simulink model "ssc_car_fuel_cell_1motor"  (R2026a)
settings: Solver=daessc  StopTime=195  FixedStep=1e-3  AbsTol=1e-3
InitFcn:
  | %Vehicle = sm_car_vehcfg_checkConfig(Vehicle);
undefined symbols (not defined in the file): Control, Driver, Init, Maneuver1, Vehicle
libraries: fl_lib x93, nesl_utility x38, GasN_lib x21, sdl_lib x10, simulink_extras x6, SimscapeFluids_lib x6, simulink x5, customMath_lib x5, slpidlib x4, ee_lib x3, autolibshared x2, sl_discontinuities x2
(part 4 of 4)

== system ssc_car_fuel_cell_1motor/Vehicle/Powertrain/FuelCell1Motor/Fuel Cell/Fuel Cell/Oxygen Source/Humidifier ==
  Desired RH : Inport
  Constant : Constant  Value=FuelCell.Humidifier.Tin.Value
  Filter : Subsystem  mask(First-order lag supporting vector signals){b=[1 1 1 1]*0.01, x_initial=[0 0 0 0]}
      mask prompts: b "Filter time constant"; x_initial "Initial output"
      mask help: Models a lag of the form 1/(b*s+1) where s is the Laplace operator.
  Gain : Gain  Gain=[0;0;0;1]
  PS-Simulink Converter : nesl_utility/PS-Simulink Converter  PhysicalDomain=network_engine_domain  SubClassName=ps_output  LeftPortType=input  RightPortType=output  PseudoPeriodic=off  Frequencies=[]  VectorFormat=1-D array  Unit=1  AffineConversion=off
  Perfect Insulator : fl_lib/Thermal/Thermal Elements/Perfect Insulator  T_specify=off  T_priority=None  T=0 K  T_nominal_specify=off  T_nominal_value=1  T_nominal_unit=K
  Pipe : GasN_lib/Pipe (N Gas)  length=FuelCell.Humidifier.xPipe.Value m  area=FuelCell.Humidifier.areaPipe.Value cm^2  Dh=FuelCell.Humidifier.dHydraulic.Value cm  extra_length=FuelCell.Humidifier.xFriction.Value m  roughness=FuelCell.Humidifier.roughness.Value m  Re_lam=FuelCell.Humidifier.laminarReynoldsMax.Value  Re_tur=FuelCell.Humidifier.turbulentReynoldsMin.Value  shape_factor=FuelCell.Humidifier.frictionDarcy.Value  Nu_lam=FuelCell.Humidifier.laminarNusselt.Value  p0=FuelCell.Humidifier.p.Value MPa  T0=FuelCell.Humidifier.T.Value degC  comp=GasN.composition_enum.mole  y0=FuelCell.Humidifier.rMoleFractions.Value'  x0=[1; 0; 0; 0]  tau_c=FuelCell.Humidifier.timeCondensation.Value s  isCond=FuelCell.Humidifier.speciesCondensed.Value'
  Simulink-PS Converter : nesl_utility/Simulink-PS Converter  PhysicalDomain=network_engine_domain  SubClassName=ps_input  LeftPortType=input  RightPortType=output  PseudoPeriodic=off  Frequencies=[]  NoiseDistribution=none  NoiseParameters=[]  Unit=1  AffineConversion=off  FilteringAndDerivatives=provide  SimscapeFilterOrder=1  InputFilterTimeConstant=0.001  UdotUserProvided=0
  Simulink-PS Converter1 : nesl_utility/Simulink-PS Converter  PhysicalDomain=network_engine_domain  SubClassName=ps_input  LeftPortType=input  RightPortType=output  PseudoPeriodic=off  Frequencies=[]  NoiseDistribution=none  NoiseParameters=[]  Unit=1  AffineConversion=off  FilteringAndDerivatives=provide  SimscapeFilterOrder=1  InputFilterTimeConstant=0.001  UdotUserProvided=0
  Simulink-PS Converter6 : nesl_utility/Simulink-PS Converter  PhysicalDomain=network_engine_domain  SubClassName=ps_input  LeftPortType=input  RightPortType=output  PseudoPeriodic=off  Frequencies=[]  NoiseDistribution=none  NoiseParameters=[]  Unit=1  AffineConversion=off  FilteringAndDerivatives=provide  SimscapeFilterOrder=1  InputFilterTimeConstant=0.001  UdotUserProvided=0
  Static Humidifier : gn_supplement_lib/Static Humidifier  Kp=0.5 kg/s
  A : PMIOPort  Side=Left
  B : PMIOPort  Port=2  Side=Right
  wires:
  Filter/1(Out) -> Simulink-PS Converter1/1
  Gain/1 -> Filter/1(In)
  PS-Simulink Converter/1 -> Gain/1
  Constant/1 -> Simulink-PS Converter/1
  Desired RH/1 -> Simulink-PS Converter6/1
  connections:
  Perfect Insulator/LConn1 -- Pipe/LConn2
  Pipe/LConn4 -- Simulink-PS Converter/RConn1
  Simulink-PS Converter1/RConn1 -- Pipe/LConn3
  PS-Simulink Converter/LConn1 -- Static Humidifier/RConn1
  Static Humidifier/LConn1 -- Simulink-PS Converter6/RConn1
  Pipe/LConn1 -- A/RConn1
  B/RConn1 -- Static Humidifier/LConn2 -- Pipe/RConn1

== system ssc_car_fuel_cell_1motor/Vehicle/Powertrain/FuelCell1Motor/Fuel Cell/Fuel Cell/ThermalMgmt/Pump Control ==
  TStack : Inport
  TRef : Inport  Port=2
  PID Controller : slpidlib/PID Controller  Controller=PID  Form=Parallel  TimeDomain=Continuous-time  UseExternalTs=off  SampleTime=-1  IntegratorMethod=Forward Euler  FilterMethod=Forward Euler  ControllerParametersSource=internal  P=FuelCell.Thermal.PumpCtrl.Kp.Value  I=FuelCell.Thermal.PumpCtrl.Ki.Value  UseKiTs=off  D=FuelCell.Thermal.PumpCtrl.Kd.Value  UseExternalDerivativeSource=off  N=FuelCell.Thermal.PumpCtrl.filter.Value  UseFilter=on  TunerSelectOption=Transfer Function Based (PID Tuner App)  ZeroCross=off  InitialConditionSource=internal  InitialConditionForIntegrator=FuelCell.Thermal.PumpCtrl.lowerlim.Value  InitialConditionForFilter=FuelCell.Thermal.PumpCtrl.lowerlim.Value  DifferentiatorICPrevScaledInput=0  ExternalReset=none  TrackingMode=off  Kt=1  LimitOutput=on  SatLimitsSource=internal  UpperSaturationLimit=FuelCell.Thermal.PumpCtrl.upperlim.Value  LowerSaturationLimit=FuelCell.Thermal.PumpCtrl.lowerlim.Value  LinearizeAsGain=on  AntiWindupMode=clamping  Kb=1  LimitIntegrator=off  UpperIntegratorSaturationLimit=inf  LowerIntegratorSaturationLimit=-inf  POutMin=[]  POutMax=[]  IOutMin=[]  IOutMax=[]  DOutMin=[]  DOutMax=[]  NOutMin=[]  NOutMax=[]  SumOutMin=[]  SumOutMax=[]  SaturationOutMin=[]  SaturationOutMax=[]  PParamMin=[]  PParamMax=[]  IParamMin=[]  IParamMax=[]  DParamMin=[]  DParamMax=[]  NParamMin=[]  NParamMax=[]  KbParamMin=[]  KbParamMax=[]  KtParamMin=[]  KtParamMax=[]  KbOutMin=[]  KbOutMax=[]  KtOutMin=[]  KtOutMax=[]  IntegratorOutMin=[]  IntegratorOutMax=[]  FilterOutMin=[]  FilterOutMax=[]  SumI1OutMin=[]  SumI1OutMax=[]  SumI2OutMin=[]  SumI2OutMax=[]  SumI3OutMin=[]  SumI3OutMax=[]  SumI4OutMin=[]  SumI4OutMax=[]  SumDOutMin=[]  SumDOutMax=[]  DifferentiatorOutMin=[]  DifferentiatorOutMax=[]  FilterDiffOutCoefMin=[]  FilterDiffOutCoefMax=[]  ReciprocalOutMin=[]  ReciprocalOutMax=[]  SumDenOutMin=[]  SumDenOutMax=[]  SumNumOutMin=[]  SumNumOutMax=[]  DivideOutMin=[]  DivideOutMax=[]  UdiffTsProdOutMin=[]  UdiffTsProdOutMax=[]  NTsProdOutMin=[]  NTsProdOutMax=[]  UintegralTsProdOutMin=[]  UintegralTsProdOutMax=[]  UngainTsProdOutMin=[]  UngainTsProdOutMax=[]  ClampingZeroOutDataTypeStr=Inherit: Inherit via back propagation  ClampingZeroOutMin=[]  ClampingZeroOutMax=[]  FilterDenConstantOutDataTypeStr=Inherit: Inherit via back propagation  FilterDenConstantOutMin=[]  FilterDenConstantOutMax=[]  PCopyOutDataTypeStr=Inherit: Inherit via back propagation  PCopyOutMin=[]  PCopyOutMax=[]  NCopyOutDataTypeStr=Inherit: Inherit via back propagation  NCopyOutMin=[]  NCopyOutMax=[]  IntegratorContinuousStateAttributes=''  IntegratorStateMustResolveToSignalObject=off  IntegratorRTWStateStorageClass=Auto  FilterContinuousStateAttributes=''  FilterStateMustResolveToSignalObject=off  FilterRTWStateStorageClass=Auto  ParallelPVariant=InternalParameters  IdealPVariant=Disabled  IVariant=InternalParameters  DVariant=InternalParameters  IntegratorVariant=Continuous  SatVariant=Enabled  AWVariant=ContClampingParallel  PCopyVariant=Disabled  TRVariant=Disabled  FdbkBlocksVariant=Forward  IdealPFdbkVariant=Disabled  SatFdbkVariant=Disabled  DerivativeFilterVariant=ContFilter  NVariant=InternalParameters  NCopyVariant=Disabled  FilterICVariant=InternalICsFilter  IntegratorICVariant=InternalICs  ExternalResetVariant=Disabled  TRSumVariant=Passthrough  SumFdbkVariant=Disabled  SumVariant=Sum_PID  TsampFilterVariant=InternalTs  TsampNgainVariant=Passthrough  TsampIntegralVariant=Disabled_SignalSpec  ExternalSaturationOutDataTypeStr=Inherit: Same as second input  DerivativeSourceVariant=ErrorSignal  PreIntVariant=InternalPreInt
  Subtract : Sum  Inputs=+-
  Transfer Fcn (with initial outputs)1 : simulink_extras/Additional Linear/Transfer Fcn (with initial outputs)  N=[1]  D="[1  1]"  Y0=.5  U0=80
  y : Outport
  wires:
  TStack/1 -> Subtract/2
  PID Controller/1 -> y/1
  TRef/1 -> Transfer Fcn (with initial outputs)1/1
  Transfer Fcn (with initial outputs)1/1 -> Subtract/1
  Subtract/1 -> PID Controller/1

== system ssc_car_fuel_cell_1motor/Vehicle/Powertrain/FuelCell1Motor/Fuel Cell/Fuel Cell/ThermalMgmt/Sensor TStack ==
  PS-Simulink Converter2 : nesl_utility/PS-Simulink Converter  PhysicalDomain=network_engine_domain  SubClassName=ps_output  LeftPortType=input  RightPortType=output  PseudoPeriodic=off  Frequencies=[]  VectorFormat=1-D array  Unit=degC  AffineConversion=on
  Temperature Sensor : fl_lib/Thermal/Thermal Sensors/Temperature Sensor  temperature_measure=foundation.enum.MeasurementReference.difference
  Thermal Reference : fl_lib/Thermal/Thermal Elements/Thermal Reference
  A : PMIOPort  Side=Left
  T : Outport
  wires:
  PS-Simulink Converter2/1 -> T/1
  connections:
  Temperature Sensor/LConn1 -- A/RConn1
  PS-Simulink Converter2/LConn1 -- Temperature Sensor/RConn2
  Thermal Reference/LConn1 -- Temperature Sensor/RConn1

== system ssc_car_fuel_cell_1motor/Vehicle/Powertrain/FuelCell1Motor/Fuel Cell/Fuel Cell/ThermalMgmt/Tank ==
  Perfect Insulator : fl_lib/Thermal/Thermal Elements/Perfect Insulator  T_specify=off  T_priority=None  T=0 K  T_nominal_specify=off  T_nominal_value=1  T_nominal_unit=K
  Tank : SimscapeFluids_lib/Thermal Liquid/Tanks & Accumulators/Tank (TL)  num_inlet=2  pressure_spec=1  tank_pressure=0.101325 MPa  volume_spec=1  tank_area=FuelCell.Thermal.Tank.area.Value cm^2  level_TLU=[0, 3, 5] m  volume_TLU=[0, 4, 6] m^3  inlet_height_A=[.1] m  inlet_area_A=[.01] m^2  inlet_heights_AB=FuelCell.Thermal.Tank.elevationAB.Value m  inlet_areas_AB=FuelCell.Thermal.Tank.areaAB.Value cm^2  inlet_heights_ABC=[.1, .05, 0] m  inlet_areas_ABC=[.01, .01, .01] m^2  inlet_heights_ABCD=linspace(0.1, 0, 4) m  inlet_areas_ABCD=0.01 * ones(1, 4) m^2  inlet_heights_ABCDE=linspace(0.1, 0, 5) m  inlet_areas_ABCDE=0.01 * ones(1, 5) m^2  inlet_heights_ABCDEF=linspace(0.1, 0, 6) m  inlet_areas_ABCDEF=0.01 * ones(1, 6) m^2  level_check=simscape.enum.assert.action.error  capacity_check=1  max_capacity=FuelCell.Thermal.Tank.volume.Value l  g=FuelCell.Thermal.Tank.g.Value m/s^2  level_specify=on  level_priority=None  level=0 m  level_nominal_specify=off  level_nominal_value=1  level_nominal_unit=m  volume_specify=on  volume_priority=High  volume=FuelCell.Thermal.Tank.volumeLiquid.Value l  volume_nominal_specify=off  volume_nominal_value=1  volume_nominal_unit=m^3  mass_specify=off  mass_priority=None  mass=5e+3 kg  mass_nominal_specify=off  mass_nominal_value=1  mass_nominal_unit=kg  T_I_specify=off  T_I_priority=High  T_I=293.15 K  T_I_nominal_specify=off  T_I_nominal_value=1  T_I_nominal_unit=K
  A : PMIOPort  Side=Right
  B : PMIOPort  Port=2  Side=Left
  connections:
  B/RConn1 -- Tank/LConn2
  Tank/LConn1 -- A/RConn1
  Tank/RConn1 -- Perfect Insulator/LConn1

== system ssc_car_fuel_cell_1motor/Vehicle/Powertrain/FuelCell1Motor/Fuel Cell/Fuel Cell/Oxygen Source/Chiller/Heat Control ==
  TDes : Inport
  Absolute Reference (N Gas) : GasN_lib/Absolute Reference (N Gas)
  PS Subtract : customMath_lib/PS Subtract
  Product M cp : customMath_lib/PS Custom Product
  Product Q : customMath_lib/PS Custom Product
  Sensor Mass Flow Rate : GasN_lib/Mass Flow Rate Sensor (N Gas)
  Sensor P T : GasN_lib/Pressure and Temperature Sensor (N Gas)
  Sensor Thermo : GasN_lib/Thermodynamic Properties Sensor (N Gas)
  Simulink-PS Converter4 : nesl_utility/Simulink-PS Converter  PhysicalDomain=network_engine_domain  SubClassName=ps_input  LeftPortType=input  RightPortType=output  PseudoPeriodic=off  Frequencies=[]  NoiseDistribution=none  NoiseParameters=[]  Unit=K  AffineConversion=off  FilteringAndDerivatives=provide  SimscapeFilterOrder=1  InputFilterTimeConstant=0.001  UdotUserProvided=0
  A : PMIOPort  Side=Left
  Q : PMIOPort  Port=2  Side=Right
  B : PMIOPort  Port=3  Side=Right
  wires:
  TDes/1 -> Simulink-PS Converter4/1
  connections:
  B/RConn1 -- Sensor Mass Flow Rate/RConn4
  Product Q/RConn1 -- Q/RConn1
  PS Subtract/LConn1 -- Simulink-PS Converter4/RConn1
  Absolute Reference (N Gas)/LConn1 -- Sensor P T/RConn3
  Product M cp/RConn1 -- Product Q/LConn1
  PS Subtract/RConn1 -- Product Q/LConn2
  Product M cp/LConn1 -- Sensor Mass Flow Rate/RConn1
  PS Subtract/LConn2 -- Sensor P T/RConn2
  Product M cp/LConn2 -- Sensor Thermo/RConn3
  Sensor Mass Flow Rate/LConn1 -- A/RConn1 -- Sensor Thermo/LConn1 -- Sensor P T/LConn1

== system ssc_car_fuel_cell_1motor/Vehicle/Powertrain/FuelCell1Motor/Fuel Cell/Fuel Cell/Oxygen Source/Humidifier/Filter ==
  In : Inport
  Gain : Gain  Gain=1./b
  Integrator : Integrator  InitialCondition=x_initial.*b
  Sum : Sum  Inputs=|+-  InputSameDT=on  SaturateOnIntegerOverflow=on  OutDataTypeStr=Inherit: Same as first input
  Out : Outport  VectorParamsAs1DForOutWhenUnconnected=off
  wires:
  Sum/1 -> Integrator/1
  In/1 -> Sum/1
  Integrator/1 -> Gain/1
  Gain/1 -> Sum/2, Out/1
